simulink model "test"  (R2019a)
settings: Solver=VariableStepAuto  StartTime=0.0  StopTime=100  MaxStep=0.01  RelTol=1e-3
settings Model: Creator=lucas  LastModifiedBy=lucas

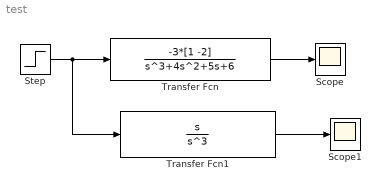
== system test ==
  Scope : Scope
  Scope1 : Scope
  Step : Step  SampleTime=0
  Transfer Fcn : TransferFcn  Numerator=-3*[1 -2]  Denominator=[1 4 5 6]
  Transfer Fcn1 : TransferFcn  Numerator=[1 0 ]  Denominator=[1 0 0 0]
  wires:
  Step/1 -> Transfer Fcn1/1, Transfer Fcn/1
  Transfer Fcn/1 -> Scope/1
  Transfer Fcn1/1 -> Scope1/1
